simulink model "evirici_1_faz"  (R2017a)
settings: Solver=ode23tb  StartTime=0.0  StopTime=0.02  RelTol=1e-3  EnableMultiTasking=on
values from neighbouring files (symbols this model uses):
  f = 1/T    (= 0.01)    [Buck_Kod.m]
undefined symbols (not defined in the file or in its folder): fider
libraries: powerlib x12, powerlib_meascontrol x1
settings Model: Creator=hp  LastModifiedBy=HCS
settings DataIOCC: LimitDataPoints=on  SaveFormat=Array  SignalLoggingSaveFormat=ModelDataLogs
settings OptimizationCC: ExpressionDepthLimit=2147483647  InitFltsAndDblsToZero=on  LifeSpan=inf
settings DebuggingCC: SaveWithParameterizedLinksMsg=none  UnderspecifiedInitializationDetection=Classic  MergeDetectMultiDrivingBlocksExec=none  SignalResolutionControl=TryResolveAllWithWarning  SolverPrmCheckMsg=warning  MultiTaskDSMMsg=warning  MultiTaskCondExecSysMsg=none  FcnCallInpInsideContextMsg=warning  StateNameClashWarn=warning  SFUnexpectedBacktrackingDiag=warning  SFNoUnconditionalDefaultTransitionDiag=warning  SFExecutionAtInitializationDiag=none
settings HardwareCC: ProdBitPerPointer=32  ProdBitPerSizeT=32  ProdBitPerPtrDiffT=32  ProdLargestAtomicFloat=None  ProdIntDivRoundTo=Undefined  ProdEndianess=Unspecified  ProdWordSize=32  ProdHWDeviceType=32-bit Generic
settings ModelReferenceCC: PropagateSignalLabelsOutOfModel=off
settings GRTTargetCC: TargetFcnLib=ansi_tfl_tmw.mat  TargetLangStandard=C89/C90 (ANSI)  CombineOutputUpdateFcns=off  GRTInterface=on
settings ConfigComp: CovMetricSettings=dw  CovSaveCumulativeToWorkspaceVar=on  CovSaveSingleToWorkspaceVar=on  CovExternalEMLEnable=off
settings SimscapeCC: SimscapeNormalizeSystem=off

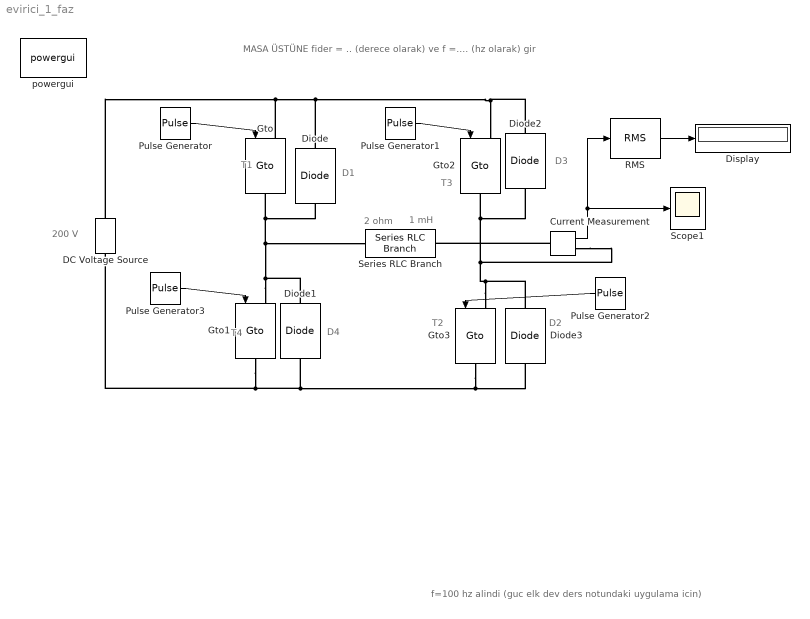
== system evirici_1_faz ==
  note: D1
  note: 1 mH
  note: 2 ohm
  note: D4
  note: D2
  note: D3
  note: MASA ÜSTÜNE
      | fider = ..  (derece olarak)    ve    f =.... (hz olarak) gir
  note: T3
  note: T1
  note: T2
  note: T4
  note: 200 V
  note: f=100 hz alindi (guc elk dev ders notundaki uygulama icin)
  Current Measurement : powerlib/Measurements/Current Measurement  PhasorSimulation=off  OutputType=Complex  PSBequivalent=0
  DC Voltage Source : powerlib/Electrical Sources/DC Voltage Source  Amplitude=200  Measurements=None
  Diode{,1..3} (4 alike) : powerlib/Power Electronics/Diode  Ron=0.000001  Lon=1e-6  Vf=0  IC=0  UseSnubber=off  Rs=1e5  Cs=inf  Measurements=off
  Display : Display
  Gto{,1..3} (4 alike) : powerlib/Power Electronics/Gto  Ron=0.00001  Lon=1e-6  Vf=0  Tf=10e-6  Tt=20e-6  IC=0  Rs=1e5  Cs=inf  Measurements=off
      settings: SourceProductBaseCode=PS
  Pulse Generator : DiscretePulseGenerator  PulseType=Time based  Period=1/f  PulseWidth=50  PhaseDelay=-(fider/360)*(1/f)
  Pulse Generator1 : DiscretePulseGenerator  PulseType=Time based  Period=1/f  PulseWidth=50  PhaseDelay=(1/f)*0.5
  Pulse Generator2 : DiscretePulseGenerator  PulseType=Time based  Period=1/f  PulseWidth=50
  Pulse Generator3 : DiscretePulseGenerator  PulseType=Time based  Period=1/f  PulseWidth=50  PhaseDelay=(1/f)*(180-fider)/360
  RMS : powerlib_meascontrol/Measurements/RMS  TrueRMS=on  Freq=f  RMSInit=2*f  Ts=0
  Scope1 : Scope
  Series RLC Branch : powerlib/Elements/Series RLC Branch  LConnTagsString=__new0  RConnTagsString=__new0  BranchType=RL  Resistance=2  Inductance=1e-3  SetiL0=off  InitialCurrent=0  Capacitance=inf  Setx0=off  InitialVoltage=0  Measurements=Branch voltage and current
  powergui : powerlib/powergui  Priority=1  SimulationMode=Discrete  SampleTime=50e-7  frequency=60  Iterations=50  frequencyindice=0  Pbase=100e6  ErrMax=1e-4  UnitsV=kV  UnitsW=MW  buscounter=0  FunctionMessages=off  echomessages=off  EnableUseOfTLC=off  CurrentSourceSwitches=off  DisableSnubberDevices=off  DisableRonSwitches=off  DisableVfSwitches=off  DisplayEquations=off  AutomaticDiscreteSolvers=off  SolverType=Tustin  Interpol=off  ExternalGateDelay=off  methode=off  Ts=0  x0status=blocks  SPID=off  SwTol=0  HookPort=off  NonlinearTolerance=1e-4  nMaxIteration=100  ContinueOnMaxIteration=off  RestoreLinks=warning  ResistiveCurrentMeasurement=off  Frange=[0:2:500]  Ylog=off  Xlog=on  ShowGrid=off  save=off  variable=ZData  structure=0  ZoomFFT=off  StartTime=0.0  cycles=1  DisplayStyle=1  fundamental=60  FreqAxis=off  MaxFrequency=1000  frequencyindicesteady=1  RmsSteady=1  display=off
  wires:
  Pulse Generator/1 -> Gto/1
  Pulse Generator3/1 -> Gto1/1
  Pulse Generator1/1 -> Gto2/1
  Pulse Generator2/1 -> Gto3/1
  Current Measurement/1 -> RMS/1, Scope1/1
  RMS/1 -> Display/1
  connections:
  Gto1/LConn1 -- Diode1/RConn1 -- Series RLC Branch/LConn1 -- Diode/LConn1 -- Gto/RConn1
  Gto3/LConn1 -- Gto2/RConn1 -- Diode2/LConn1 -- Current Measurement/RConn1 -- Diode3/RConn1
  Gto3/RConn1 -- Diode3/LConn1 -- Diode1/LConn1 -- Gto1/RConn1 -- DC Voltage Source/LConn1
  Current Measurement/LConn1 -- Series RLC Branch/RConn1
  DC Voltage Source/RConn1 -- Diode2/RConn1 -- Gto2/LConn1 -- Diode/RConn1 -- Gto/LConn1
